simulink model "RocketPlantWithActuatorController"  (R2025b)
settings: Solver=VariableStepAuto  StartTime=0.0  StopTime=10  RelTol=1e-3
model workspace (MAT data in the model file):
  controller_mode : controller_modes (value not decoded)
settings Model: Creator=karadeli  LastModifiedBy=Kaan Kalkandelen

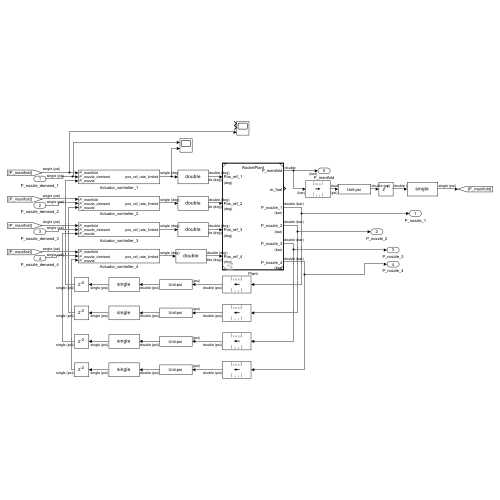
[thumbnail: Simulink's stored preview of the top-level diagram]
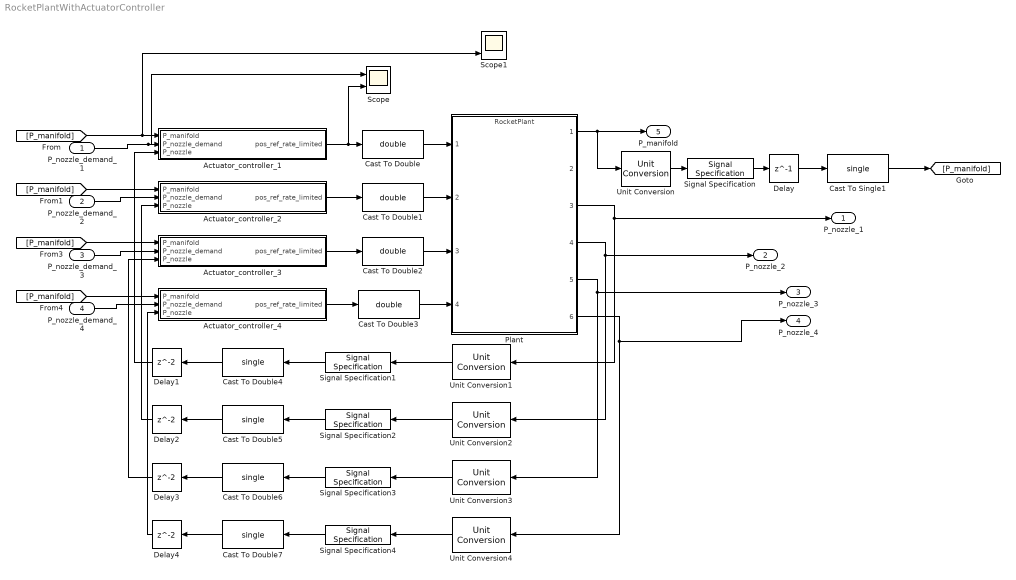
== system RocketPlantWithActuatorController ==
  P_nozzle_demand_1 : Inport
  P_nozzle_demand_2 : Inport  Port=2
  P_nozzle_demand_3 : Inport  Port=3
  P_nozzle_demand_4 : Inport  Port=4
  Actuator_controller_1 : Subsystem
  Actuator_controller_2 : Subsystem
  Actuator_controller_3 : Subsystem
  Actuator_controller_4 : Subsystem
  Cast To Double{,1..3} (4 alike) : DataTypeConversion  OutDataTypeStr=double  SaturateOnIntegerOverflow=off  RndMeth=Floor
  Cast To Double{4..7} (4 alike) : DataTypeConversion  OutDataTypeStr=single  SaturateOnIntegerOverflow=off  RndMeth=Floor
  Cast To Single1 : DataTypeConversion  OutDataTypeStr=single  SaturateOnIntegerOverflow=off  RndMeth=Floor
  Delay : Delay  DelayLength=1
  Delay{1..4} (4 alike) : Delay
  Plant : ModelReference  ModelNameDialog=RocketPlant.slx  SimulationMode=Normal  ModelReferenceVersion=1.28
  Scope : Scope  NumInputPorts=2
      settings: ActiveDisplayYMinimum=-96.281661987304659  ActiveDisplayYMaximum=866.53495788574219
  Scope1 : Scope  NumInputPorts=3
      settings: ActiveDisplayYMinimum=-543.89154052734364  ActiveDisplayYMaximum=4895.0238647460938  DataLoggingVariableName=ScopeData2
  Signal Specification{,1..4} (5 alike) : SignalSpecification  Unit=psi
  Unit Conversion{,1..4} (5 alike) : UnitConversion
  P_nozzle_1 : Outport
  P_nozzle_2 : Outport  Port=2
  P_nozzle_3 : Outport  Port=3
  P_nozzle_4 : Outport  Port=4
  P_manifold : Outport  Port=5
  wires:
  Plant/1 -> P_manifold/1, Unit Conversion/1
  Delay/1 -> Cast To Single1/1
  [P_manifold] -> Scope1/3, Actuator_controller_1/1(P_manifold)
  Actuator_controller_2/1(pos_ref_rate_limited) -> Cast To Double1/1
  Actuator_controller_3/1(pos_ref_rate_limited) -> Cast To Double2/1
  Actuator_controller_4/1(pos_ref_rate_limited) -> Cast To Double3/1
  [P_manifold] -> Actuator_controller_2/1(P_manifold)
  [P_manifold] -> Actuator_controller_4/1(P_manifold)
  [P_manifold] -> Actuator_controller_3/1(P_manifold)
  Cast To Double/1 -> Plant/1
  Cast To Double1/1 -> Plant/2
  Cast To Double2/1 -> Plant/3
  Cast To Double3/1 -> Plant/4
  Cast To Single1/1 -> [P_manifold]
  P_nozzle_demand_1/1 -> Scope/1, Actuator_controller_1/2(P_nozzle_demand)
  P_nozzle_demand_2/1 -> Actuator_controller_2/2(P_nozzle_demand)
  P_nozzle_demand_3/1 -> Actuator_controller_3/2(P_nozzle_demand)
  P_nozzle_demand_4/1 -> Actuator_controller_4/2(P_nozzle_demand)
  Actuator_controller_1/1(pos_ref_rate_limited) -> Scope/2, Cast To Double/1
  Unit Conversion/1 -> Signal Specification/1
  Signal Specification/1 -> Delay/1
  Delay1/1 -> Actuator_controller_1/3(P_nozzle)
  Unit Conversion1/1 -> Signal Specification1/1
  Cast To Double4/1 -> Delay1/1
  Signal Specification1/1 -> Cast To Double4/1
  Signal Specification2/1 -> Cast To Double5/1
  Cast To Double5/1 -> Delay2/1
  Unit Conversion2/1 -> Signal Specification2/1
  Unit Conversion4/1 -> Signal Specification4/1
  Cast To Double7/1 -> Delay4/1
  Signal Specification4/1 -> Cast To Double7/1
  Signal Specification3/1 -> Cast To Double6/1
  Cast To Double6/1 -> Delay3/1
  Unit Conversion3/1 -> Signal Specification3/1
  Delay2/1 -> Actuator_controller_2/3(P_nozzle)
  Delay3/1 -> Actuator_controller_3/3(P_nozzle)
  Delay4/1 -> Actuator_controller_4/3(P_nozzle)
  Plant/3 -> P_nozzle_1/1, Unit Conversion1/1
  Plant/4 -> P_nozzle_2/1, Unit Conversion2/1
  Plant/6 -> P_nozzle_4/1, Unit Conversion4/1
  Plant/5 -> Unit Conversion3/1, P_nozzle_3/1

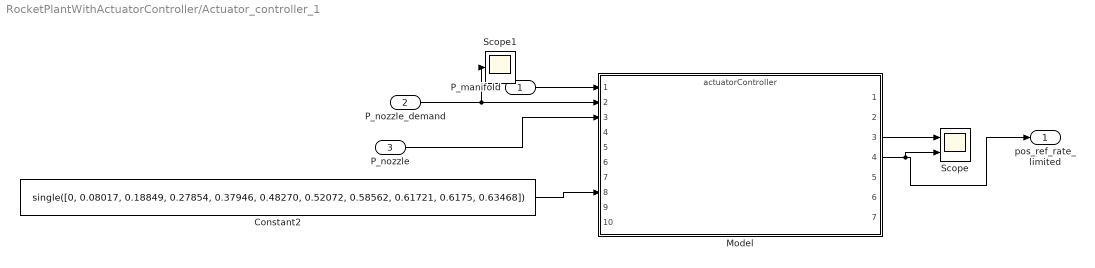
== system RocketPlantWithActuatorController/Actuator_controller_1 ==
  P_manifold : Inport
  P_nozzle_demand : Inport  Port=2
  P_nozzle : Inport  Port=3
  Constant2 : Constant  Value=single([0, 0.08017, 0.18849, 0.27854, 0.37946, 0.48270, 0.52072, 0.58562, 0.61721, 0.6175, 0.63468])  OutDataTypeStr=single
  Model : ModelReference  ModelNameDialog=actuatorController.slx  SimulationMode=Normal  ModelReferenceVersion=1.74
  Scope : Scope  NumInputPorts=2
      settings: ActiveDisplayYMinimum=-134.99999999999997  ActiveDisplayYMaximum=1215
  Scope1 : Scope
      settings: ActiveDisplayYMinimum=-1  ActiveDisplayYMaximum=1  DataLoggingVariableName=ScopeData3
  pos_ref_rate_limited : Outport
  wires:
  Model/4 -> Scope/2, pos_ref_rate_limited/1
  P_nozzle_demand/1 -> Scope1/1, Model/2
  P_manifold/1 -> Model/1
  Model/3 -> Scope/1
  P_nozzle/1 -> Model/3
  Constant2/1 -> Model/8

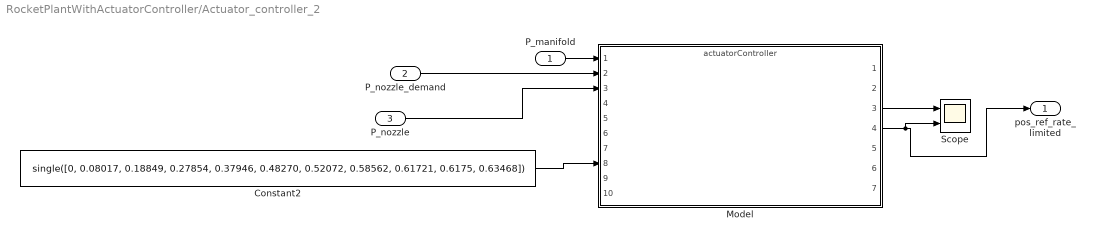
== system RocketPlantWithActuatorController/Actuator_controller_2 ==
  P_manifold : Inport
  P_nozzle_demand : Inport  Port=2
  P_nozzle : Inport  Port=3
  Constant2 : Constant  Value=single([0, 0.08017, 0.18849, 0.27854, 0.37946, 0.48270, 0.52072, 0.58562, 0.61721, 0.6175, 0.63468])  OutDataTypeStr=single
  Model : ModelReference  ModelNameDialog=actuatorController.slx  SimulationMode=Normal  ModelReferenceVersion=1.74
  Scope : Scope  NumInputPorts=2
      settings: ActiveDisplayYMinimum=-134.99999999999997  ActiveDisplayYMaximum=1215
  pos_ref_rate_limited : Outport
  wires:
  Constant2/1 -> Model/8
  P_nozzle/1 -> Model/3
  Model/3 -> Scope/1
  P_manifold/1 -> Model/1
  P_nozzle_demand/1 -> Model/2
  Model/4 -> pos_ref_rate_limited/1, Scope/2

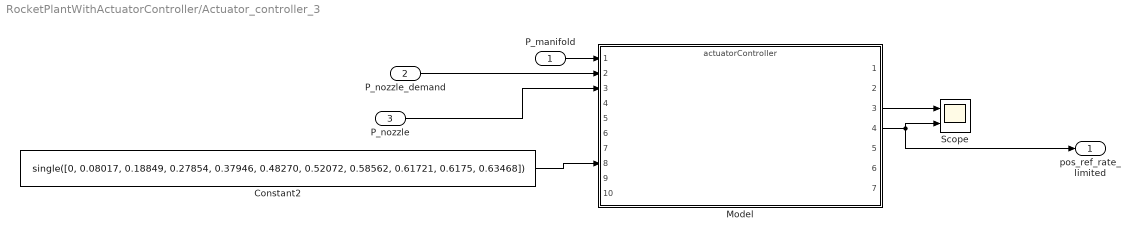
== system RocketPlantWithActuatorController/Actuator_controller_3 ==
  P_manifold : Inport
  P_nozzle_demand : Inport  Port=2
  P_nozzle : Inport  Port=3
  Constant2 : Constant  Value=single([0, 0.08017, 0.18849, 0.27854, 0.37946, 0.48270, 0.52072, 0.58562, 0.61721, 0.6175, 0.63468])  OutDataTypeStr=single
  Model : ModelReference  ModelNameDialog=actuatorController.slx  SimulationMode=Normal  ModelReferenceVersion=1.74
  Scope : Scope  NumInputPorts=2
      settings: ActiveDisplayYMinimum=-134.99999999999997  ActiveDisplayYMaximum=1215
  pos_ref_rate_limited : Outport
  wires:
  Model/4 -> Scope/2, pos_ref_rate_limited/1
  P_nozzle_demand/1 -> Model/2
  P_manifold/1 -> Model/1
  Model/3 -> Scope/1
  P_nozzle/1 -> Model/3
  Constant2/1 -> Model/8

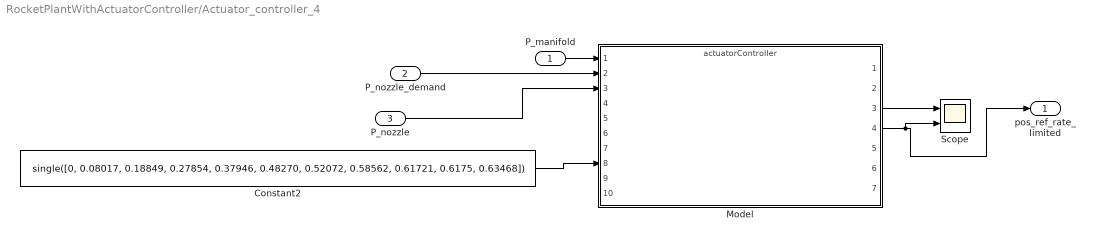
== system RocketPlantWithActuatorController/Actuator_controller_4 ==
  P_manifold : Inport
  P_nozzle_demand : Inport  Port=2
  P_nozzle : Inport  Port=3
  Constant2 : Constant  Value=single([0, 0.08017, 0.18849, 0.27854, 0.37946, 0.48270, 0.52072, 0.58562, 0.61721, 0.6175, 0.63468])  OutDataTypeStr=single
  Model : ModelReference  ModelNameDialog=actuatorController.slx  SimulationMode=Normal  ModelReferenceVersion=1.74
  Scope : Scope  NumInputPorts=2
      settings: ActiveDisplayYMinimum=-134.99999999999997  ActiveDisplayYMaximum=1215
  pos_ref_rate_limited : Outport
  wires:
  Constant2/1 -> Model/8
  P_nozzle/1 -> Model/3
  Model/3 -> Scope/1
  P_manifold/1 -> Model/1
  P_nozzle_demand/1 -> Model/2
  Model/4 -> pos_ref_rate_limited/1, Scope/2
